simulink model "thermal_model_simulink"  (R2025b)
settings: Solver=VariableStepAuto  StartTime=0.0  StopTime=10.0  RelTol=1e-3
values from neighbouring files (symbols this model uses):
  C1 = 50    [task1.m]
  C2 = 60    [task1.m]
  q_amp = 3    [task1.m]
  R12 = (p.R1 * p.R2) / (p.R1 + p.R2)    [app.m]    (also in task1.m = 5)
  R2 = 10    [task1.m]
  R23 = (p.R2 * p.R3) / (p.R2 + p.R3)    [app.m]    (also in task1.m = 5)
  t_step = 600    [task1.m]
settings Model: Creator=jhosh  LastModifiedBy=jhosh
settings DataIOCC: ReturnWorkspaceOutputsName=simOut

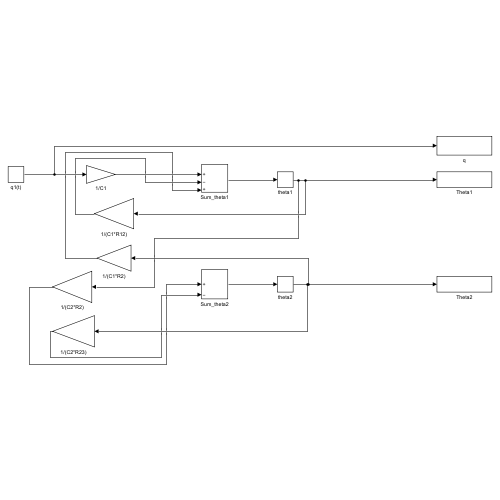
[thumbnail: Simulink's stored preview of the top-level diagram]
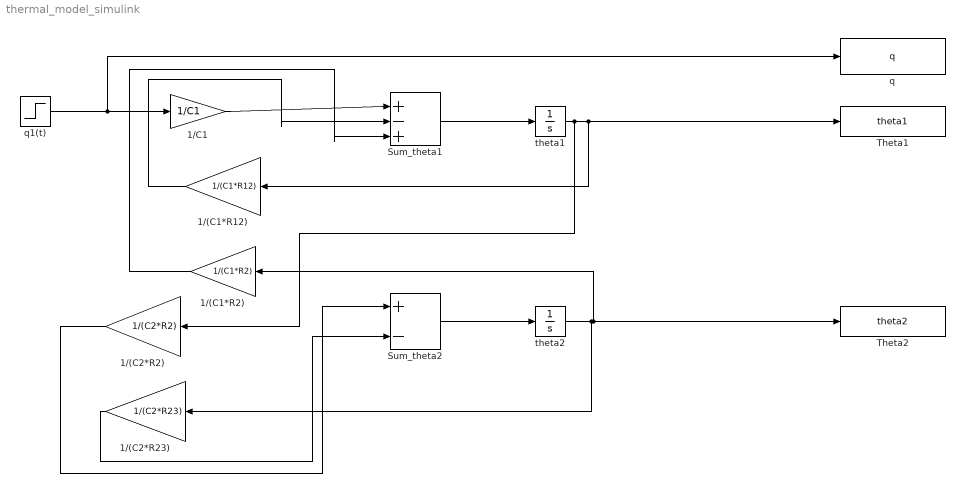
== system thermal_model_simulink ==
  1/(C1*R12) : Gain  Gain=1/(C1*R12)
  1/(C1*R2) : Gain  Gain=1/(C1*R2)
  1/(C2*R2) : Gain  Gain=1/(C2*R2)
  1/(C2*R23) : Gain  Gain=1/(C2*R23)
  1/C1 : Gain  Gain=1/C1
  Sum_theta1 : Sum  Inputs=|+-+
  Sum_theta2 : Sum  Inputs=|+-
  Theta1 : ToWorkspace  VariableName=theta1  SaveFormat=Timeseries  SampleTime=-1
  Theta2 : ToWorkspace  VariableName=theta2  SaveFormat=Timeseries  SampleTime=-1
  q : ToWorkspace  VariableName=q  SaveFormat=Timeseries  SampleTime=-1
  q1(t) : Step  Time=t_step  After=q_amp  SampleTime=0
  theta1 : Integrator
  theta2 : Integrator
  wires:
  q1(t)/1 -> q/1, 1/C1/1
  1/C1/1 -> Sum_theta1/1
  Sum_theta1/1 -> theta1/1
  theta1/1 -> Theta1/1, 1/(C1*R12)/1, 1/(C2*R2)/1
  Sum_theta2/1 -> theta2/1
  theta2/1 -> 1/(C1*R2)/1, Theta2/1, 1/(C2*R23)/1
  1/(C1*R12)/1 -> Sum_theta1/2
  1/(C1*R2)/1 -> Sum_theta1/3
  1/(C2*R23)/1 -> Sum_theta2/2
  1/(C2*R2)/1 -> Sum_theta2/1
